simulink model "affineManeuver"  (Simulink 7.5)
settings: Solver=ode4  StartTime=0.0  StopTime=10.0  FixedStep=0.01  MaxStep=0.02  RelTol=1e-3
values from neighbouring files (symbols this model uses):
  dim = 2    [main.m]
  nodenum = size(P,1)    [main.m]
  stepsize = 0.005    [main.m]
  v_init = zeros(dim*nodenum,1)    [main.m]
  x_init = p+[0 0     0 0     0 0     1 1     0 1     -1 1     -2 -1]'    [main.m]
settings Model: Creator=Shiyu Zhao  LastModifiedBy=uos
settings CodeAppCC: CustomSymbolStrType=$N$R$M_T

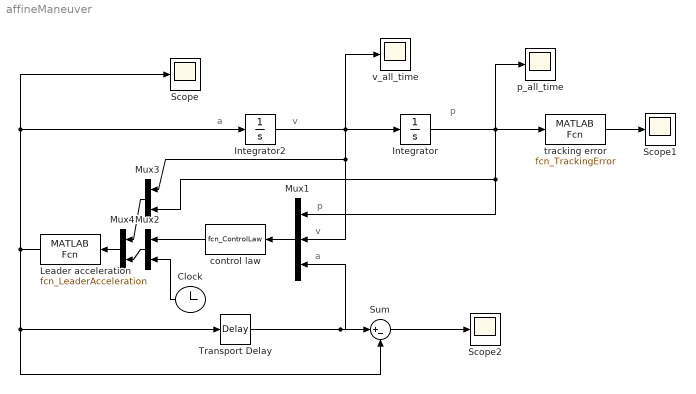
== system affineManeuver ==
  note: a
  note: p
  note: v
  note: p
  note: v
  note: a
  Clock : Clock
      settings: Decimation=10
  Integrator : Integrator  InitialCondition=x_init
  Integrator2 : Integrator  InitialCondition=v_init
  Leader acceleration : MATLABFcn  MATLABFcn=fcn_LeaderAcceleration
  Mux1 : Mux  Inputs=3
  Mux2 : Mux  Inputs=2
  Mux3 : Mux  Inputs=2
  Mux4 : Mux  Inputs=2
  Scope : Scope
      settings: SaveName=a_all
  Scope1 : Scope
      settings: SaveName=error_all
  Scope2 : Scope
      settings: SaveName=aDiff_all
  Sum : Sum  Inputs=|+-  OutDataType=fixdt(1, 16)  OutScaling=2^0
  Transport Delay : TransportDelay  DelayTime=stepsize  InitialOutput=zeros(dim*nodenum,1)
  control law : MATLABFcn  MATLABFcn=fcn_ControlLaw
  p_all_time : Scope
      settings: SaveName=p_all_time
  tracking error : MATLABFcn  MATLABFcn=fcn_TrackingError
  v_all_time : Scope
      settings: SaveName=v_all_time
  wires:
  tracking error/1 -> Scope1/1
  Mux1/1 -> control law/1
  Integrator/1 -> tracking error/1, p_all_time/1, Mux1/1, Mux3/2
  Integrator2/1 -> Integrator/1, v_all_time/1, Mux1/2, Mux3/1
  control law/1 -> Mux2/1
  Clock/1 -> Mux2/2
  Leader acceleration/1 -> Integrator2/1, Scope/1, Sum/2, Transport Delay/1
  Transport Delay/1 -> Mux1/3, Sum/1
  Sum/1 -> Scope2/1
  Mux3/1 -> Mux4/1
  Mux2/1 -> Mux4/2
  Mux4/1 -> Leader acceleration/1
